simulink model "Adruino_Model"  (R2024a)
settings: Solver=VariableStepAuto  StartTime=0.0  StopTime=10.0  RelTol=1e-3
settings Model: Creator=BVM  LastModifiedBy=BVM

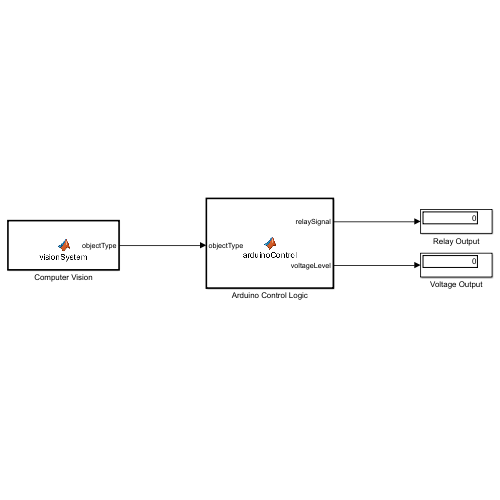
[thumbnail: Simulink's stored preview of the top-level diagram]
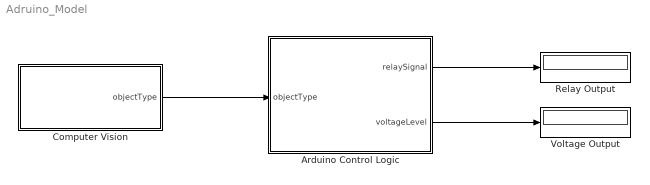
== system Adruino_Model ==
  Arduino Control Logic : MATLAB Function  TreatAsAtomicUnit=on
  Computer Vision : MATLAB Function  TreatAsAtomicUnit=on
  Relay Output : Display
  Voltage Output : Display
  wires:
  Arduino Control Logic/1(relaySignal) -> Relay Output/1
  Arduino Control Logic/2(voltageLevel) -> Voltage Output/1
  Computer Vision/1(objectType) -> Arduino Control Logic/1(objectType)

== matlab function Adruino_Model/Computer Vision ==
  data: objectType output
function objectType = visionSystem()
% Simulate object detection logic
% Output: objectType (1 = Human, 2 = Large Animal, 3 = Small Animal)
    objectType = randi([1, 3]); % Randomly simulates detection of different objects
end

== matlab function Adruino_Model/Arduino Control Logic ==
  data: objectType input; relaySignal output; voltageLevel output
function [relaySignal, voltageLevel] = arduinoControl(objectType)
% Simulate Arduino control logic based on detected object
% Input: objectType (1 = Human, 2 = Large Animal, 3 = Small Animal)
% Output: relaySignal (0 or 1), voltageLevel (0, 5, or 12)

    if objectType == 1
        relaySignal = 0; % Deactivate relay for human
        voltageLevel = 0; % No voltage
    elseif objectType == 2
        relaySignal = 1; % Activate relay
        voltageLevel = 12; % High voltage for large animals
    else
        relaySignal = 1; % Activate relay
        voltageLevel = 5; % Lower voltage for small animals
    end
end
